simulink model "NDI"  (R2022a)
settings: Solver=ode4  StartTime=0  StopTime=100  FixedStep=fcs.Ts  RelTol=1e-3
undefined symbols (not defined in the file or in its folder): Aactuator, ac, AeroCoeff, ControlAllocation, DUmax, DUmin, EngineTable, F, fcs, ft, g, hground, IC, kg, LandingGear, Light, m, MIL, Mode_deflection_aileron, Mode_deflection_elevator, Mode_deflection_rudder, Mode_deflection_TVC_y, Mode_deflection_TVC_z, N, Ninv_2nozzle, Ninv_no_nozzle, PIController, s, Sensor, sigbuilder_block, slug, state0, sysID_DAQ, sysID_OBES, Umax_2nozzle, Umax_no_nozzle, Umin_2nozzle, Umin_no_nozzle, WMM2020
libraries: aerolibconvert2 x31, slpidlib x11, simulink x6, sharedutil x4, aerolibatmos2 x3, aerolibwind2 x3, aerolibbdyn x3, aerolibgravity2 x2, sharedtransform x1
(part 3 of 13)

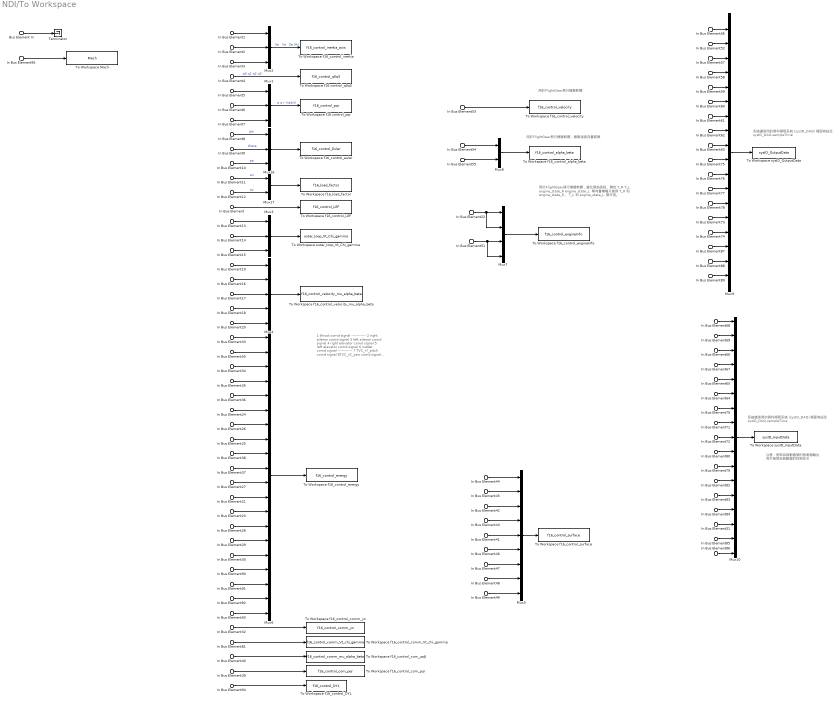
== system NDI/To Workspace ==
  note: 系統識別用的資料擷取系統 (sysID_DAQ)
      | 裡面有設定 sysID_DAQ.sampleTime
  note: 1 thrust comd signal
      | -----------
      | 2 right aileron comd signal
      | 3 left aileron comd signal
      | 4 right elevator comd signal
      | 5 left elevator comd signal
      | 6 rudder comd signal
      | -----------
      | 7 TVC_rY_pitch comd signal
      | 8TVC_rZ_yaw comd signal
      | 9 TVC_lY_pitch comd signal
      | 10TVC_lZ_yaw comd signal
      |
      | 11 thrust signal
      | -----------
      | 12 right aileron signal
      | 13 left aileron signal
      | 14 right elevator signal
      | 15 left elevator signal
      | 16 rudder signal
      | -----------
      | 17 TVC_rY_pitch signal
      | 18 TVC_rZ_yaw signal
      | 19 TVC_lY_pitch signal
      | 20 TVC_lZ_yaw signal
  note: 用於FlightGear飛行模擬軟體
  note: 用於FlightGear飛行模擬軟體，繪製速度向量箭頭
  note: 用於FlightGear飛行模擬軟體，變化尾焰長短、顏色
      | T_R
      | T_L
      | engine_state_R
      | engine_state_L
      |
      | 單向量噴嘴只使用 T_R 和 engine_state_R。
      | T_L 和 engine_state_L 無作用。
  note: 注意：是取自致動器號的感測器輸出
      | 而不是取自致動器的控制命令
  note: 系統識別用的資料擷取系統 (sysID_DAQ)
      | 裡面有設定 sysID_DAQ.sampleTime
  In Bus Element1 : Inport  PortName=PlantData  Element=npos
  In Bus Element2 : Inport  PortName=PlantData  Element=epos
  In Bus Element3 : Inport  PortName=PlantData  Element=altitude
  In Bus Element4 : Inport  PortName=PlantData  Element=q0q1q2q3
  In Bus Element5 : Inport  PortName=PlantData  Element=p
  In Bus Element61 : Inport  PortName=PlantData  Element=p
  In Bus Element6 : Inport  PortName=PlantData  Element=q
  In Bus Element62 : Inport  PortName=PlantData  Element=q
  In Bus Element7 : Inport  PortName=PlantData  Element=r
  In Bus Element63 : Inport  PortName=PlantData  Element=r
  In Bus Element8 : Inport  PortName=PlantData  Element=phi
  In Bus Element58 : Inport  PortName=PlantData  Element=phi
  In Bus Element9 : Inport  PortName=PlantData  Element=theta
  In Bus Element59 : Inport  PortName=PlantData  Element=theta
  In Bus Element10 : Inport  PortName=PlantData  Element=psi
  In Bus Element60 : Inport  PortName=PlantData  Element=psi
  In Bus Element11 : Inport  PortName=PlantData  Element=an
  In Bus Element12 : Inport  PortName=PlantData  Element=ay
  In Bus Element : Inport  PortName=PlantData  Element=AeroActBus.LEF_deg
  In Bus Element80 : Inport  PortName=PlantData  Element=AeroActBus.LEF_deg
  In Bus Element30 : Inport  PortName=PlantData  Element=AeroActBus.Rudder_deg
  In Bus Element41 : Inport  PortName=PlantData  Element=AeroActBus.Rudder_deg
  In Bus Element65 : Inport  PortName=PlantData  Element=AeroActBus.Rudder_deg
  In Bus Element21 : Inport  PortName=PlantData  Element=AeroActBus.right Aileron_deg
  In Bus Element42 : Inport  PortName=PlantData  Element=AeroActBus.right Aileron_deg
  In Bus Element66 : Inport  PortName=PlantData  Element=AeroActBus.right Aileron_deg
  In Bus Element23 : Inport  PortName=PlantData  Element=AeroActBus.left Aileron_deg
  In Bus Element43 : Inport  PortName=PlantData  Element=AeroActBus.left Aileron_deg
  In Bus Element67 : Inport  PortName=PlantData  Element=AeroActBus.left Aileron_deg
  In Bus Element28 : Inport  PortName=PlantData  Element=AeroActBus.right Elevator_deg
  In Bus Element44 : Inport  PortName=PlantData  Element=AeroActBus.right Elevator_deg
  In Bus Element68 : Inport  PortName=PlantData  Element=AeroActBus.right Elevator_deg
  In Bus Element29 : Inport  PortName=PlantData  Element=AeroActBus.left Elevator_deg
  In Bus Element45 : Inport  PortName=PlantData  Element=AeroActBus.left Elevator_deg
  In Bus Element69 : Inport  PortName=PlantData  Element=AeroActBus.left Elevator_deg
  In Bus Element79 : Inport  PortName=PlantData  Element=AeroActBus.SB_deg
  In Bus Element{13,19,53,56} (4 alike) : Inport  PortName=PlantData  Element=Vt
  In Bus Element14 : Inport  PortName=PlantData  Element=chi
  In Bus Element88 : Inport  PortName=PlantData  Element=chi
  In Bus Element15 : Inport  PortName=PlantData  Element=gamma
  In Bus Element20 : Inport  PortName=PlantData  Element=gamma
  In Bus Element89 : Inport  PortName=PlantData  Element=gamma
  In Bus Element16 : Inport  PortName=PlantData  Element=alpha
  In Bus Element54 : Inport  PortName=PlantData  Element=alpha
  In Bus Element52 : Inport  PortName=PlantData  Element=alpha
  In Bus Element17 : Inport  PortName=PlantData  Element=beta
  In Bus Element55 : Inport  PortName=PlantData  Element=beta
  In Bus Element57 : Inport  PortName=PlantData  Element=beta
  In Bus Element18 : Inport  PortName=PlantData  Element=mu
  In Bus Element87 : Inport  PortName=PlantData  Element=mu
  In Bus Element33 : Inport  PortName=PlantData  Element=fadec_cmd.thrust
  In Bus Element25 : Inport  PortName=PlantData  Element=fadec_cmd.TVC_rz
  In Bus Element26 : Inport  PortName=PlantData  Element=fadec_cmd.TVC_ry
  In Bus Element37 : Inport  PortName=PlantData  Element=fadec_cmd.TVC_lz
  In Bus Element38 : Inport  PortName=PlantData  Element=fadec_cmd.TVC_ly
  In Bus Element24 : Inport  PortName=PlantData  Element=fcs_cmd.rudder
  In Bus Element34 : Inport  PortName=PlantData  Element=fcs_cmd.left aileron
  In Bus Element35 : Inport  PortName=PlantData  Element=fcs_cmd.right elevator
  In Bus Element36 : Inport  PortName=PlantData  Element=fcs_cmd.left elevator
  In Bus Element50 : Inport  PortName=PlantData  Element=fcs_cmd.right aileron
  In Bus Element27 : Inport  PortName=PlantData  Element=PropBus.T
  In Bus Element22 : Inport  PortName=PlantData  Element=PropBus.T
  In Bus Element51 : Inport  PortName=PlantData  Element=PropBus.engine_state
  In Bus Element82 : Inport  PortName=PlantData  Element=PropBus.Tx
  In Bus Element83 : Inport  PortName=PlantData  Element=PropBus.Ty
  In Bus Element84 : Inport  PortName=PlantData  Element=PropBus.Tz
  In Bus Element73 : Inport  PortName=PlantData  Element=ay_offset
  In Bus Element74 : Inport  PortName=PlantData  Element=az_offset
  In Bus Element75 : Inport  PortName=PlantData  Element=p_dot
  In Bus Element76 : Inport  PortName=PlantData  Element=q_dot
  In Bus Element77 : Inport  PortName=PlantData  Element=r_dot
  In Bus Element85 : Inport  PortName=PlantData  Element=f
  In Bus Element86 : Inport  PortName=PlantData  Element=N
  In Bus Element90 : Inport  PortName=PlantData  Element=PropActBus.TVC_ry_pitch_deg
  In Bus Element46 : Inport  PortName=PlantData  Element=PropActBus.TVC_ry_pitch_deg
  In Bus Element64 : Inport  PortName=PlantData  Element=PropActBus.TVC_ry_pitch_deg
  In Bus Element91 : Inport  PortName=PlantData  Element=PropActBus.TVC_rz_yaw_deg
  In Bus Element47 : Inport  PortName=PlantData  Element=PropActBus.TVC_rz_yaw_deg
  In Bus Element70 : Inport  PortName=PlantData  Element=PropActBus.TVC_rz_yaw_deg
  In Bus Element92 : Inport  PortName=PlantData  Element=PropActBus.TVC_ly_pitch_deg
  In Bus Element48 : Inport  PortName=PlantData  Element=PropActBus.TVC_ly_pitch_deg
  In Bus Element71 : Inport  PortName=PlantData  Element=PropActBus.TVC_ly_pitch_deg
  In Bus Element93 : Inport  PortName=PlantData  Element=PropActBus.TVC_lz_yaw_deg
  In Bus Element49 : Inport  PortName=PlantData  Element=PropActBus.TVC_lz_yaw_deg
  In Bus Element72 : Inport  PortName=PlantData  Element=PropActBus.TVC_lz_yaw_deg
  In Bus Element78 : Inport  PortName=PlantData  Element=ax_offset
  In Bus Element32 : Inport  PortName=PlantData  Element=LogDataBus.cmd_yz
  In Bus Element39 : Inport  PortName=PlantData  Element=LogDataBus.cmd_pqr
  In Bus Element40 : Inport  PortName=PlantData  Element=LogDataBus.cmd_mu_alpha_beta
  In Bus Element81 : Inport  PortName=PlantData  Element=LogDataBus.cmd_Vt_chi_gamma
  In Bus Element94 : Inport  PortName=PlantData  Element=LogDataBus.drag_sideForce_lift
  Bus Element In : Inport  Port=2  PortName=EnvData
  In Bus Element31 : Inport  Port=2  PortName=EnvData  Element=qbar
  In Bus Element95 : Inport  Port=2  PortName=EnvData  Element=Mach
  Mux{1..3,16} (4 alike) : Mux  Inputs=3
  Mux10 : Mux  Inputs=17
  Mux17 : Mux  Inputs=2
  Mux4 : Mux  Inputs=5
  Mux5 : Mux  Inputs=9
  Mux6 : Mux  Inputs=20
  Mux7 : Mux
  Mux8 : Mux  Inputs=2
  Mux9 : Mux  Inputs=18
  Terminator : Terminator
  To Workspace Mach : ToWorkspace  VariableName=Mach  SaveFormat=Timeseries  SampleTime=-1
  To Workspace f16 control_pqr : ToWorkspace  VariableName=f16_control_pqr  SaveFormat=Timeseries  SampleTime=-1
  To Workspace f16 control_q0q3 : ToWorkspace  VariableName=f16_control_q0q3  SaveFormat=Timeseries  SampleTime=-1
  To Workspace f16_control_DYL : ToWorkspace  VariableName=f16_control_DYL  SaveFormat=Timeseries  SampleTime=-1
  To Workspace f16_control_LEF : ToWorkspace  VariableName=f16_control_LEF  SaveFormat=Timeseries  SampleTime=-1
  To Workspace f16_control_alpha_beta : ToWorkspace  VariableName=f16_control_alpha_beta  SaveFormat=Timeseries  SampleTime=-1
  To Workspace f16_control_com_pqr : ToWorkspace  VariableName=f16_control_com_pqr  SaveFormat=Timeseries  SampleTime=-1
  To Workspace f16_control_com_μαβ : ToWorkspace  VariableName=f16_control_comm_mu_alpha_beta  SaveFormat=Timeseries  SampleTime=-1
  To Workspace f16_control_comm_Vt_chi_gamma : ToWorkspace  VariableName=f16_control_comm_Vt_chi_gamma  SaveFormat=Timeseries  SampleTime=-1
  To Workspace f16_control_comm_yz : ToWorkspace  VariableName=f16_control_comm_yz  SaveFormat=Timeseries  SampleTime=-1
  To Workspace f16_control_energy : ToWorkspace  VariableName=f16_control_energy  SaveFormat=Timeseries  SampleTime=-1
  To Workspace f16_control_engineInfo : ToWorkspace  VariableName=f16_control_engineInfo  SaveFormat=Timeseries  SampleTime=-1
  To Workspace f16_control_euler : ToWorkspace  VariableName=f16_control_Euler  SaveFormat=Timeseries  SampleTime=-1
  To Workspace f16_control_inertia : ToWorkspace  VariableName=f16_control_inertia_axis  SaveFormat=Timeseries  SampleTime=-1
      settings: Save2DSignal=2-D array (concatenate along first dimension)
  To Workspace f16_control_surface : ToWorkspace  VariableName=f16_control_surface  SaveFormat=Timeseries  SampleTime=-1
  To Workspace f16_control_velocity : ToWorkspace  VariableName=f16_control_velocity  SaveFormat=Timeseries  SampleTime=-1
  To Workspace f16_control_velocity_mu_alpha_beta : ToWorkspace  VariableName=f16_control_velocity_mu_alpha_beta  SaveFormat=Timeseries  SampleTime=-1
  To Workspace f16_load_factor : ToWorkspace  VariableName=f16_load_factor  SaveFormat=Timeseries  SampleTime=-1
  To Workspace outer_loop_Vt_Chi_gamma : ToWorkspace  VariableName=outer_loop_Vt_Chi_gamma  SaveFormat=Timeseries  SampleTime=-1
  To Workspace sysID_InputData : ToWorkspace  VariableName=sysID_InputData  SaveFormat=Timeseries  SampleTime=sysID_DAQ.sampleTime
  To Workspace sysID_OutputData : ToWorkspace  VariableName=sysID_OutputData  SaveFormat=Timeseries  SampleTime=sysID_DAQ.sampleTime
  wires:
  Mux2/1 -> To Workspace f16_control_inertia/1  "Xe   Ye   Ze (ft)"
  Mux16/1 -> To Workspace f16_control_euler/1
  In Bus Element9/1 -> Mux16/2  "theta"
  In Bus Element10/1 -> Mux16/3  "psi"
  In Bus Element4/1 -> To Workspace f16 control_q0q3/1  "q0 q1 q2 q3"
  In Bus Element11/1 -> Mux17/1  "an"
  In Bus Element8/1 -> Mux16/1  "phi"
  Mux17/1 -> To Workspace f16_load_factor/1
  In Bus Element12/1 -> Mux17/2  "ay"
  Mux1/1 -> To Workspace f16 control_pqr/1  "p q r (rad/s)"
  In Bus Element5/1 -> Mux1/1
  In Bus Element6/1 -> Mux1/2
  In Bus Element7/1 -> Mux1/3
  In Bus Element1/1 -> Mux2/1
  In Bus Element2/1 -> Mux2/2
  In Bus Element3/1 -> Mux2/3
  In Bus Element/1 -> To Workspace f16_control_LEF/1
  In Bus Element13/1 -> Mux3/1
  In Bus Element14/1 -> Mux3/2
  In Bus Element15/1 -> Mux3/3
  Mux3/1 -> To Workspace outer_loop_Vt_Chi_gamma/1
  In Bus Element19/1 -> Mux4/1
  In Bus Element16/1 -> Mux4/2
  In Bus Element17/1 -> Mux4/3
  In Bus Element18/1 -> Mux4/4
  In Bus Element20/1 -> Mux4/5
  Mux4/1 -> To Workspace f16_control_velocity_mu_alpha_beta/1
  Mux6/1 -> To Workspace f16_control_energy/1
  Bus Element In/1 -> Terminator/1
  In Bus Element33/1 -> Mux6/1
  In Bus Element50/1 -> Mux6/2
  In Bus Element34/1 -> Mux6/3
  In Bus Element35/1 -> Mux6/4
  In Bus Element36/1 -> Mux6/5
  In Bus Element24/1 -> Mux6/6
  In Bus Element27/1 -> Mux6/11
  In Bus Element21/1 -> Mux6/12
  In Bus Element23/1 -> Mux6/13
  In Bus Element28/1 -> Mux6/14
  In Bus Element29/1 -> Mux6/15
  In Bus Element30/1 -> Mux6/16
  In Bus Element90/1 -> Mux6/17
  In Bus Element91/1 -> Mux6/18
  In Bus Element92/1 -> Mux6/19
  In Bus Element93/1 -> Mux6/20
  In Bus Element41/1 -> Mux5/5
  In Bus Element47/1 -> Mux5/7
  In Bus Element49/1 -> Mux5/9
  In Bus Element48/1 -> Mux5/8
  In Bus Element46/1 -> Mux5/6
  In Bus Element44/1 -> Mux5/1
  In Bus Element45/1 -> Mux5/2
  In Bus Element42/1 -> Mux5/3
  In Bus Element43/1 -> Mux5/4
  Mux5/1 -> To Workspace f16_control_surface/1
  In Bus Element26/1 -> Mux6/7
  In Bus Element25/1 -> Mux6/8
  In Bus Element38/1 -> Mux6/9
  In Bus Element37/1 -> Mux6/10
  Mux8/1 -> To Workspace f16_control_alpha_beta/1
  In Bus Element53/1 -> To Workspace f16_control_velocity/1
  In Bus Element55/1 -> Mux8/2
  In Bus Element54/1 -> Mux8/1
  Mux7/1 -> To Workspace f16_control_engineInfo/1
  In Bus Element22/1 -> Mux7/2, Mux7/1
  In Bus Element51/1 -> Mux7/4, Mux7/3
  In Bus Element78/1 -> Mux9/13
  In Bus Element65/1 -> Mux10/5
  In Bus Element75/1 -> Mux9/10
  In Bus Element80/1 -> Mux10/10
  In Bus Element52/1 -> Mux9/2
  In Bus Element79/1 -> Mux10/11
  In Bus Element59/1 -> Mux9/5
  In Bus Element62/1 -> Mux9/8
  In Bus Element83/1 -> Mux10/13
  In Bus Element73/1 -> Mux9/14
  In Bus Element71/1 -> Mux10/8
  In Bus Element60/1 -> Mux9/6
  In Bus Element61/1 -> Mux9/7
  In Bus Element68/1 -> Mux10/1
  In Bus Element77/1 -> Mux9/12
  In Bus Element66/1 -> Mux10/3
  In Bus Element72/1 -> Mux10/9
  In Bus Element69/1 -> Mux10/2
  In Bus Element70/1 -> Mux10/7
  In Bus Element63/1 -> Mux9/9
  In Bus Element58/1 -> Mux9/4
  In Bus Element57/1 -> Mux9/3
  In Bus Element86/1 -> Mux10/17
  In Bus Element67/1 -> Mux10/4
  In Bus Element88/1 -> Mux9/17
  In Bus Element85/1 -> Mux10/16
  In Bus Element76/1 -> Mux9/11
  In Bus Element84/1 -> Mux10/14
  In Bus Element31/1 -> Mux10/15
  In Bus Element82/1 -> Mux10/12
  In Bus Element87/1 -> Mux9/16
  In Bus Element74/1 -> Mux9/15
  In Bus Element89/1 -> Mux9/18
  In Bus Element64/1 -> Mux10/6
  Mux10/1 -> To Workspace sysID_InputData/1
  In Bus Element56/1 -> Mux9/1
  Mux9/1 -> To Workspace sysID_OutputData/1
  In Bus Element94/1 -> To Workspace f16_control_DYL/1
  In Bus Element81/1 -> To Workspace f16_control_comm_Vt_chi_gamma/1
  In Bus Element32/1 -> To Workspace f16_control_comm_yz/1
  In Bus Element40/1 -> To Workspace f16_control_com_μαβ/1
  In Bus Element39/1 -> To Workspace f16_control_com_pqr/1
  In Bus Element95/1 -> To Workspace Mach/1

== system NDI/Environment/Dynamic Pressure ==
  Vt : Inport
  rho : Inport  Port=2
  1/2rhoV^2 : Gain  Gain=1/2  SaturateOnIntegerOverflow=on  OutDataTypeStr=Inherit: Same as input  ParamDataTypeStr=Inherit: Same as input
  Product2 : Product  InputSameDT=on  SaturateOnIntegerOverflow=on  OutDataTypeStr=Inherit: Same as first input
  Square : Math  Operator=square  SignedPower=on
  qbar : Outport
  wires:
  rho/1 -> Product2/2
  Square/1 -> Product2/1
  1/2rhoV^2/1 -> qbar/1
  Product2/1 -> 1/2rhoV^2/1
  Vt/1 -> Square/1

== system NDI/Environment/ISP  ==
  note: 1 T
      | 2 a (Speed of sound)
      | 3 P
      | 4 rho
      | 5 g
      | 6 mu (Coefficient of viscosity)
  h(m) : Inport
  Demux : Demux  Outputs=[1,1,1,1,1,1]
      settings: DisplayOption=none
  MATLAB Function : MATLAB Function  TreatAsAtomicUnit=on
  end8 : Terminator
  end9 : Terminator
  T (K) : Outport  VectorParamsAs1DForOutWhenUnconnected=off
  a (m/s) : Outport  Port=2  VectorParamsAs1DForOutWhenUnconnected=off
  P (HPa) : Outport  Port=3  VectorParamsAs1DForOutWhenUnconnected=off
  rho (kg/m^3) : Outport  Port=4  VectorParamsAs1DForOutWhenUnconnected=off
  wires:
  MATLAB Function/1(ISP_output) -> Demux/1
  h(m)/1 -> MATLAB Function/1(h)
  Demux/4 -> rho (kg/m^3)/1  "rho(kg/m^3)"
  Demux/2 -> a (m/s)/1  "a(m/s)"
  Demux/1 -> T (K)/1  "T(K)"
  Demux/5 -> end8/1  "g (m/s^2)"
  Demux/6 -> end9/1  "mu"
  Demux/3 -> P (HPa)/1  "P(Pa)"

== system NDI/Environment/Mach Number ==
  Vt : Inport
  a : Inport  Port=2
  Product1 : Product  Inputs=*/  InputSameDT=on  SaturateOnIntegerOverflow=on  OutDataTypeStr=Inherit: Same as first input
  Mach : Outport  Unit=1  VectorParamsAs1DForOutWhenUnconnected=off
  wires:
  Vt/1 -> Product1/1
  a/1 -> Product1/2
  Product1/1 -> Mach/1

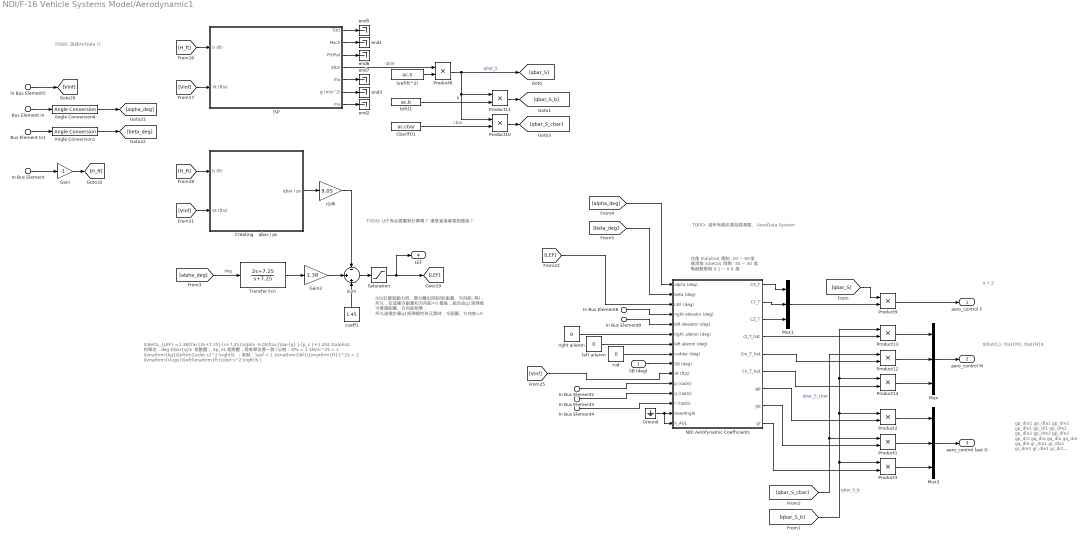
== system NDI/F-16 Vehicle Systems Model/Aerodynamic1 ==
  note: NDI計算氣動力時，要分離出控制項(副翼、方向舵..等)，
      | 所以，在這裡令副翼和方向舵=0
      | 最後，組合成g1矩陣後 才會跟副翼、方向舵相乘，
      | 所以這裡計算g1矩陣裡的各元素時，令副翼、方向舵=0
  note: TODO: LEF有必要重新計算嗎？
      | 還是直接拿感測器值？
  note: X
      | Y
      | Z
  note: $\delta_{LEF} =1.38\frac{2s+7.25}{s+7.25}\alpha -9.05\frac{\bar{q} }{p_s }+1.45$
      | $\alpha$ 的單位：deg
      | $\bar{q}$ 是動壓， $p_s$ 是靜壓，兩者單位要一致 (公制：1Pa = 1 $N/m^2$ = 1 $\mathrm{kg}/\left(m{\cdot s}^2 \right)$ ；英制：1psf = 1 $\mathrm{lbf}/{\mathrm{ft}}^2$ = 1 $\mathrm{slugs}/\left(\mathrm{ft}\cdot s^2 \right)$ )
  note: $\hat{L}, \hat{M}, \hat{N}$
  note: TODO: 這所有資訊源自感測器、
      | AeroData System
  note: TODO: 改成AirData !?
  note: 攻角 $\alpha$ 限制 -20 ~ 90度
      | 側滑角 $\beta$ 限制 -30 ~ 30 度
      | 馬赫數限制 0.1 ~ 0.6 度
  note: gp_dra1
      | gp_dla1
      | gp_dre1
      | gp_dle1
      | gp_dr1
      | gp_dra2
      | gp_dla2
      | gp_dre2
      | gp_dle2
      | gp_dr2
      |
      | gq_dra
      | gq_dla
      | gq_dre
      | gq_dle
      |
      | gr_dra1
      | gr_dla1
      | gr_dre1
      | gr_dle1
      | gr_dr1
      | gr_dra2
      | gr_dla2
      | gr_dre2
      | gr_dle2
      | gr_dr2
  SB (deg) : Inport  Unit=deg
  In Bus Element : Inport  Port=2  PortName=PlantData  Element=altitude
  In Bus Element8 : Inport  Port=2  PortName=PlantData  Element=AeroActBus.right Elevator_deg
  In Bus Element9 : Inport  Port=2  PortName=PlantData  Element=AeroActBus.left Elevator_deg
  In Bus Element2 : Inport  Port=2  PortName=PlantData  Element=p
  In Bus Element3 : Inport  Port=2  PortName=PlantData  Element=q
  In Bus Element4 : Inport  Port=2  PortName=PlantData  Element=r
  In Bus Element5 : Inport  Port=2  PortName=PlantData  Element=Vt
  Bus Element In : Inport  Port=3  PortName=AirData  Element=alpha
  Bus Element In1 : Inport  Port=3  PortName=AirData  Element=beta
  Angle Conversion1 : aerolibconvert2/Angle Conversion  IU=rad  OU=deg
  Angle Conversion4 : aerolibconvert2/Angle Conversion  IU=rad  OU=deg
  Cbar(ft)1 : Constant  Value=ac.cbar
  Creating    qbar / ps : Subsystem
  Gain : Gain  Gain=-1
  Gain2 : Gain  Gain=1.38  SaturateOnIntegerOverflow=on  OutDataTypeStr=Inherit: Same as input  ParamDataTypeStr=Inherit: Same as input
  Ground : Ground
  "ISP " : Subsystem
  Mux : Mux  Inputs=3
  Mux1 : Mux  Inputs=3
  Mux3 : Mux  Inputs=3
  NDI Aerofynamic Coefficients : Subsystem
  Product{1..3,6,9..14} (10 alike) : Product
  Saturation : Saturate  UpperLimit=Aactuator.LEF.AngleLimitUpper  LowerLimit=Aactuator.LEF.AngleLimitLower
  Sref(ft^2) : Constant  Value=ac.S
  Sum : Sum  Inputs=-|+|+  InputSameDT=on  SaturateOnIntegerOverflow=on  OutDataTypeStr=Inherit: Same as first input
  Transfer Fcn : TransferFcn  Numerator=[2 7.25]  Denominator=[1 7.25]
  b(ft)1 : Constant  Value=ac.b
  coeff1 : Constant  Value=1.45
  end{1..3,5..7} (6 alike) : Terminator
  left aileron : Constant  Value=0
  r2d6 : Gain  Gain=9.05  SaturateOnIntegerOverflow=on  OutDataTypeStr=Inherit: Same as input  ParamDataTypeStr=Inherit: Same as input
  right aileron : Constant  Value=0
  rud : Constant  Value=0
  aero_control F : Outport  VectorParamsAs1DForOutWhenUnconnected=off
  aero_control M : Outport  Port=2  VectorParamsAs1DForOutWhenUnconnected=off
  aero_control fast G : Outport  Port=3  VectorParamsAs1DForOutWhenUnconnected=off
  LEF : Outport  Port=4
  wires:
  [Vinf] -> "ISP "/2(Vt (ft/s))
  "ISP "/2("Mach ") -> end1/1
  "ISP "/7(mu) -> end2/1
  "ISP "/6(g (m/s^2)) -> end3/1
  "ISP "/5(rho) -> end7/1
  "ISP "/4("qbar ") -> Product6/1  "qbar"
  "ISP "/3(P(HPa)) -> end6/1
  "ISP "/1(T(K)) -> end5/1
  r2d6/1 -> Sum/1
  Creating    qbar / ps/1(qbar / ps) -> r2d6/1
  [alpha_deg] -> Transfer Fcn/1  "deg"
  [Vinf] -> Creating    qbar / ps/2(Vt (ft/s))
  coeff1/1 -> Sum/3
  [H_ft] -> Creating    qbar / ps/1(h (ft))
  [H_ft] -> "ISP "/1(h (ft))
  Sum/1 -> Saturation/1
  Saturation/1 -> LEF/1, [LEF]
  Transfer Fcn/1 -> Gain2/1
  In Bus Element/1 -> Gain/1
  Gain/1 -> [H_ft]
  Cbar(ft)1/1 -> Product10/2  "cbar"
  b(ft)1/1 -> Product11/2  "b"
  Sref(ft^2)/1 -> Product6/2
  Product10/1 -> [qbar_S_cbar]
  Product6/1 -> Product11/1, Product10/1, [qbar_S]  "qbar_S"
  Product11/1 -> [qbar_S_b]
  [qbar_S] -> Product9/1
  Product9/1 -> aero_control F/1
  Product12/1 -> Mux/2
  Product13/1 -> Mux/1
  Product14/1 -> Mux/3
  Mux/1 -> aero_control M/1
  NDI Aerofynamic Coefficients/4(Cl_T_hat) -> Product13/2
  NDI Aerofynamic Coefficients/5(Cm_T_hat) -> Product12/2
  NDI Aerofynamic Coefficients/6(Cn_T_hat) -> Product14/2
  NDI Aerofynamic Coefficients/1(CX_T) -> Mux1/1
  NDI Aerofynamic Coefficients/2(CY_T) -> Mux1/2
  NDI Aerofynamic Coefficients/3(CZ_T) -> Mux1/3
  Mux1/1 -> Product9/2
  [qbar_S_b] -> Product13/1, Product14/1, Product2/1, Product3/1  "qbar_S_b"
  Product3/1 -> Mux3/3
  Product1/1 -> Mux3/2
  Product2/1 -> Mux3/1
  NDI Aerofynamic Coefficients/7(gp) -> Product2/2
  [qbar_S_cbar] -> Product12/1, Product1/1  "qbar_S_cbar"
  NDI Aerofynamic Coefficients/9(gr) -> Product3/2
  NDI Aerofynamic Coefficients/8(gq) -> Product1/2
  Mux3/1 -> aero_control fast G/1
  [Vinf] -> NDI Aerofynamic Coefficients/10(Vt (ft/s))
  SB (deg)/1 -> NDI Aerofynamic Coefficients/9(SB (deg))
  [LEF] -> NDI Aerofynamic Coefficients/3(LEF (deg))
  [beta_deg] -> NDI Aerofynamic Coefficients/2(beta (deg))
  [alpha_deg] -> NDI Aerofynamic Coefficients/1(alpha (deg))
  In Bus Element2/1 -> NDI Aerofynamic Coefficients/11(p (rad/s))
  In Bus Element3/1 -> NDI Aerofynamic Coefficients/12(q (rad/s))
  In Bus Element4/1 -> NDI Aerofynamic Coefficients/13(r (rad/s))
  Ground/1 -> NDI Aerofynamic Coefficients/14(GearAngle), NDI Aerofynamic Coefficients/15(h_AGL)
  Gain2/1 -> Sum/2
  Bus Element In/1 -> Angle Conversion4/1
  Angle Conversion4/1 -> [alpha_deg]
  Angle Conversion1/1 -> [beta_deg]
  Bus Element In1/1 -> Angle Conversion1/1
  In Bus Element5/1 -> [Vinf]
  In Bus Element8/1 -> NDI Aerofynamic Coefficients/4(right elevator (deg))
  In Bus Element9/1 -> NDI Aerofynamic Coefficients/5(left elevator (deg))
  right aileron/1 -> NDI Aerofynamic Coefficients/6(right alieron (deg))
  left aileron/1 -> NDI Aerofynamic Coefficients/7(left alieron (deg))
  rud/1 -> NDI Aerofynamic Coefficients/8(rudder (deg))

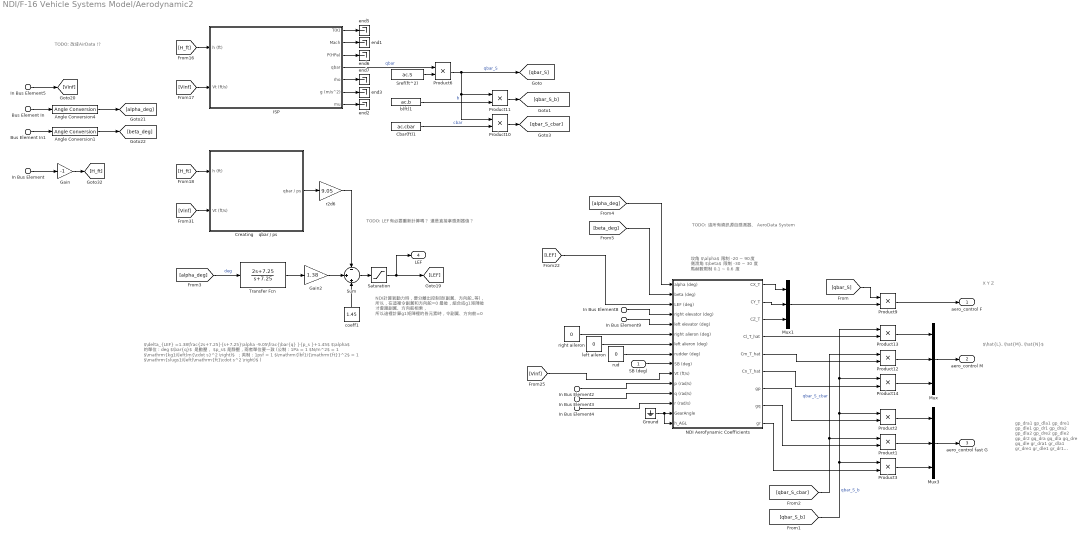
== system NDI/F-16 Vehicle Systems Model/Aerodynamic2 ==
  note: NDI計算氣動力時，要分離出控制項(副翼、方向舵..等)，
      | 所以，在這裡令副翼和方向舵=0
      | 最後，組合成g1矩陣後 才會跟副翼、方向舵相乘，
      | 所以這裡計算g1矩陣裡的各元素時，令副翼、方向舵=0
  note: TODO: LEF有必要重新計算嗎？
      | 還是直接拿感測器值？
  note: X
      | Y
      | Z
  note: $\delta_{LEF} =1.38\frac{2s+7.25}{s+7.25}\alpha -9.05\frac{\bar{q} }{p_s }+1.45$
      | $\alpha$ 的單位：deg
      | $\bar{q}$ 是動壓， $p_s$ 是靜壓，兩者單位要一致 (公制：1Pa = 1 $N/m^2$ = 1 $\mathrm{kg}/\left(m{\cdot s}^2 \right)$ ；英制：1psf = 1 $\mathrm{lbf}/{\mathrm{ft}}^2$ = 1 $\mathrm{slugs}/\left(\mathrm{ft}\cdot s^2 \right)$ )
  note: $\hat{L}, \hat{M}, \hat{N}$
  note: TODO: 這所有資訊源自感測器、
      | AeroData System
  note: TODO: 改成AirData !?
  note: 攻角 $\alpha$ 限制 -20 ~ 90度
      | 側滑角 $\beta$ 限制 -30 ~ 30 度
      | 馬赫數限制 0.1 ~ 0.6 度
  note: gp_dra1
      | gp_dla1
      | gp_dre1
      | gp_dle1
      | gp_dr1
      | gp_dra2
      | gp_dla2
      | gp_dre2
      | gp_dle2
      | gp_dr2
      |
      | gq_dra
      | gq_dla
      | gq_dre
      | gq_dle
      |
      | gr_dra1
      | gr_dla1
      | gr_dre1
      | gr_dle1
      | gr_dr1
      | gr_dra2
      | gr_dla2
      | gr_dre2
      | gr_dle2
      | gr_dr2
  SB (deg) : Inport  Unit=deg
  In Bus Element : Inport  Port=2  PortName=PlantData  Element=altitude
  In Bus Element8 : Inport  Port=2  PortName=PlantData  Element=AeroActBus.right Elevator_deg
  In Bus Element9 : Inport  Port=2  PortName=PlantData  Element=AeroActBus.left Elevator_deg
  In Bus Element2 : Inport  Port=2  PortName=PlantData  Element=p
  In Bus Element3 : Inport  Port=2  PortName=PlantData  Element=q
  In Bus Element4 : Inport  Port=2  PortName=PlantData  Element=r
  In Bus Element5 : Inport  Port=2  PortName=PlantData  Element=Vt
  Bus Element In : Inport  Port=3  PortName=AirData  Element=alpha
  Bus Element In1 : Inport  Port=3  PortName=AirData  Element=beta
  Angle Conversion1 : aerolibconvert2/Angle Conversion  IU=rad  OU=deg
  Angle Conversion4 : aerolibconvert2/Angle Conversion  IU=rad  OU=deg
  Cbar(ft)1 : Constant  Value=ac.cbar
  Creating    qbar / ps : Subsystem
  Gain : Gain  Gain=-1
  Gain2 : Gain  Gain=1.38  SaturateOnIntegerOverflow=on  OutDataTypeStr=Inherit: Same as input  ParamDataTypeStr=Inherit: Same as input
  Ground : Ground
  "ISP " : Subsystem
  Mux : Mux  Inputs=3
  Mux1 : Mux  Inputs=3
  Mux3 : Mux  Inputs=3
  NDI Aerofynamic Coefficients : Subsystem
  Product{1..3,6,9..14} (10 alike) : Product
  Saturation : Saturate  UpperLimit=Aactuator.LEF.AngleLimitUpper  LowerLimit=Aactuator.LEF.AngleLimitLower
  Sref(ft^2) : Constant  Value=ac.S
  Sum : Sum  Inputs=-|+|+  InputSameDT=on  SaturateOnIntegerOverflow=on  OutDataTypeStr=Inherit: Same as first input
  Transfer Fcn : TransferFcn  Numerator=[2 7.25]  Denominator=[1 7.25]
  b(ft)1 : Constant  Value=ac.b
  coeff1 : Constant  Value=1.45
  end{1..3,5..7} (6 alike) : Terminator
  left aileron : Constant  Value=0
  r2d6 : Gain  Gain=9.05  SaturateOnIntegerOverflow=on  OutDataTypeStr=Inherit: Same as input  ParamDataTypeStr=Inherit: Same as input
  right aileron : Constant  Value=0
  rud : Constant  Value=0
  aero_control F : Outport  VectorParamsAs1DForOutWhenUnconnected=off
  aero_control M : Outport  Port=2  VectorParamsAs1DForOutWhenUnconnected=off
  aero_control fast G : Outport  Port=3  VectorParamsAs1DForOutWhenUnconnected=off
  LEF : Outport  Port=4
  wires:
  [Vinf] -> "ISP "/2(Vt (ft/s))
  "ISP "/2("Mach ") -> end1/1
  "ISP "/7(mu) -> end2/1
  "ISP "/6(g (m/s^2)) -> end3/1
  "ISP "/5(rho) -> end7/1
  "ISP "/4("qbar ") -> Product6/1  "qbar"
  "ISP "/3(P(HPa)) -> end6/1
  "ISP "/1(T(K)) -> end5/1
  r2d6/1 -> Sum/1
  Creating    qbar / ps/1(qbar / ps) -> r2d6/1
  [alpha_deg] -> Transfer Fcn/1  "deg"
  [Vinf] -> Creating    qbar / ps/2(Vt (ft/s))
  coeff1/1 -> Sum/3
  [H_ft] -> Creating    qbar / ps/1(h (ft))
  [H_ft] -> "ISP "/1(h (ft))
  Sum/1 -> Saturation/1
  Saturation/1 -> LEF/1, [LEF]
  Transfer Fcn/1 -> Gain2/1
  In Bus Element/1 -> Gain/1
  Gain/1 -> [H_ft]
  Cbar(ft)1/1 -> Product10/2  "cbar"
  b(ft)1/1 -> Product11/2  "b"
  Sref(ft^2)/1 -> Product6/2
  Product10/1 -> [qbar_S_cbar]
  Product6/1 -> Product11/1, Product10/1, [qbar_S]  "qbar_S"
  Product11/1 -> [qbar_S_b]
  [qbar_S] -> Product9/1
  Product9/1 -> aero_control F/1
  Product12/1 -> Mux/2
  Product13/1 -> Mux/1
  Product14/1 -> Mux/3
  Mux/1 -> aero_control M/1
  NDI Aerofynamic Coefficients/4(Cl_T_hat) -> Product13/2
  NDI Aerofynamic Coefficients/5(Cm_T_hat) -> Product12/2
  NDI Aerofynamic Coefficients/6(Cn_T_hat) -> Product14/2
  NDI Aerofynamic Coefficients/1(CX_T) -> Mux1/1
  NDI Aerofynamic Coefficients/2(CY_T) -> Mux1/2
  NDI Aerofynamic Coefficients/3(CZ_T) -> Mux1/3
  Mux1/1 -> Product9/2
  [qbar_S_b] -> Product13/1, Product14/1, Product2/1, Product3/1  "qbar_S_b"
  Product3/1 -> Mux3/3
  Product1/1 -> Mux3/2
  Product2/1 -> Mux3/1
  NDI Aerofynamic Coefficients/7(gp) -> Product2/2
  [qbar_S_cbar] -> Product12/1, Product1/1  "qbar_S_cbar"
  NDI Aerofynamic Coefficients/9(gr) -> Product3/2
  NDI Aerofynamic Coefficients/8(gq) -> Product1/2
  Mux3/1 -> aero_control fast G/1
  [Vinf] -> NDI Aerofynamic Coefficients/10(Vt (ft/s))
  SB (deg)/1 -> NDI Aerofynamic Coefficients/9(SB (deg))
  [LEF] -> NDI Aerofynamic Coefficients/3(LEF (deg))
  [beta_deg] -> NDI Aerofynamic Coefficients/2(beta (deg))
  [alpha_deg] -> NDI Aerofynamic Coefficients/1(alpha (deg))
  In Bus Element2/1 -> NDI Aerofynamic Coefficients/11(p (rad/s))
  In Bus Element3/1 -> NDI Aerofynamic Coefficients/12(q (rad/s))
  In Bus Element4/1 -> NDI Aerofynamic Coefficients/13(r (rad/s))
  Ground/1 -> NDI Aerofynamic Coefficients/14(GearAngle), NDI Aerofynamic Coefficients/15(h_AGL)
  Gain2/1 -> Sum/2
  Bus Element In/1 -> Angle Conversion4/1
  Angle Conversion4/1 -> [alpha_deg]
  Angle Conversion1/1 -> [beta_deg]
  Bus Element In1/1 -> Angle Conversion1/1
  In Bus Element5/1 -> [Vinf]
  In Bus Element8/1 -> NDI Aerofynamic Coefficients/4(right elevator (deg))
  In Bus Element9/1 -> NDI Aerofynamic Coefficients/5(left elevator (deg))
  right aileron/1 -> NDI Aerofynamic Coefficients/6(right alieron (deg))
  left aileron/1 -> NDI Aerofynamic Coefficients/7(left alieron (deg))
  rud/1 -> NDI Aerofynamic Coefficients/8(rudder (deg))

== system NDI/F-16 Vehicle Systems Model/Iteration Algorithm V chi gamma ==
  note: TODO: 這有必要嗎？
      | 設定限制範圍錯誤似乎會造成計算問題，第0秒模擬失敗
  note: $\mu_c ={\mathrm{tan}}^{-1} {\left(\frac{mV_T {\chi^˙ }_{des} \mathrm{cos}\gamma-f\mathrm{sin}\chi }{mV_T {\gamma^˙ }_{des} +mg\mathrm{cos}\gamma-N\mathrm{cos}\gamma-f\mathrm{cos}\chi\mathrm{sin}\gamma }\right)}$
  note: $\alpha_c ={\mathrm{tan}}^{-1} {\left(\frac{-L+mV_T {\chi^˙ }_{des} \mathrm{cos}\gamma \mathrm{sin}\mu_c +mV_T {\gamma^˙ }_{des} \mathrm{cos}\mu_c +mg\mathrm{cos}\gamma \mathrm{cos}\mu_c-N\mathrm{cos}\mu_c\mathrm{cos}\gamma-f(\mathrm{sin}\mu_c\mathrm{sin}\chi+\mathrm{cos}\mu_c\mathrm{cos}\chi\mathrm{sin}\gamma) }{m{\dot{V} }_{T_{des} } +D+mg\mathrm{sin}\gamma-N\mathrm{sin}\gamma+f\mathrm{cos}\chi\mathrm{sin}\gamma }\right)}$
  note: $T_c =\frac{1}{\mathrm{cos}\alpha_c }{\left(m{\dot{V} }_{T_{des} } +D+mg\mathrm{sin}\gamma-N\mathrm{sin}\gamma+f\mathrm{cos}\chi\mathrm{sin}\gamma \right)}$
  note: m
  note: chi
  note: f,0,N
  note: chi
  note: f,0,N
  note: chi
  note: f,0,N
  alpha_c : Inport
  aero F : Inport  Port=2
  Vt,chi,gamma dot desire : Inport  Port=3
  beta_cmd : Inport  Port=4
  LGxyz : Inport  Port=5
  gravity : Inport  Port=6
  In Bus Element4 : Inport  Port=7  PortName=AirData  Element=Vt
  In Bus Element5 : Inport  Port=7  PortName=AirData  Element=gamma
  In Bus Element1 : Inport  Port=8  PortName=PlantData  Element=chi
  Drag_c : Fcn  Expr=-u(4)*cos(u(2))*cos(u(3))-u(5)*sin(u(3))-u(6)*sin(u(2))*cos(u(3))
  Lift_c : Fcn  Expr=u(4)*sin(u(2))-u(6)*cos(u(2))
  Mux : Mux  Inputs=7
  Mux1 : Mux
  Mux2 : Mux  Inputs=7
  Mux{3..6} (4 alike) : Mux  Inputs=2
  Mux7 : Mux  Inputs=7
  Saturation : Saturate  UpperLimit=deg2rad(90)  LowerLimit=deg2rad(-20)
  Thrust_c function : Fcn  Expr=(u(8)*u(1)+u(6)+u(8)*u(9)*sin(u(5))+u(14)*sin(u(5))-u(12)*cos(u(11))*sin(u(5)))/(cos(u(10)))
  To Workspace : ToWorkspace  VariableName=Drag_c_Lift_c  SaveFormat=Timeseries  SampleTime=-1
  alpha_c function : Fcn  Expr=atan2((-u(9)+u(10)*u(6)*cos(u(7))*sin(u(4))*u(2)+u(10)*u(6)*cos(u(4))*u(3)+u(10)*u(11)*cos(u(7))*cos(u(4))+u(15)*cos(u(4))*cos(u(7))+u(13)*(sin(u(4))*sin(u(12))+cos(u(4))*cos(u(12))*sin(u(7)))),(u(10)*u(1)+u(8)+u(10)*u(11)*sin(u(7))+u(15)*sin(u(7))-u(13)*cos(u(12))*sin(u(7))))
  mass (slugs) : Constant  Value=ac.m
  mu_c : Fcn  Expr=atan2((u(7)*u(4)*u(2)*cos(u(5))-u(9)*sin(u(8))),(u(7)*u(4)*u(3)+u(7)*u(6)*cos(u(5))-u(11)*cos(u(5))-u(9)*cos(u(8))*sin(u(5))))
  thrust_command : Outport  VectorParamsAs1DForOutWhenUnconnected=off
  mu_command : Outport  Port=2  VectorParamsAs1DForOutWhenUnconnected=off
  alpha_command : Outport  Port=3  VectorParamsAs1DForOutWhenUnconnected=off
  beta_command : Outport  Port=4  VectorParamsAs1DForOutWhenUnconnected=off
  wires:
  Vt,chi,gamma dot desire/1 -> Mux/1, Mux2/1, Mux7/1  "Vt,chi,gamma dot desire"
  In Bus Element4/1 -> Mux6/1, Mux1/1, Mux/2  "Vt"
  In Bus Element5/1 -> Mux6/2, Mux/3  "gamma"
  Mux/1 -> mu_c/1
  gravity/1 -> Mux5/2, Mux/4  "g"
  mu_c/1 -> Mux4/1, mu_command/1  "mu_c"
  aero F/1 -> Mux1/4  "X,Y,Z"
  beta_cmd/1 -> Mux4/2, Mux1/3, beta_command/1  "beta_c"
  alpha_c/1 -> Mux1/2  "alpha_c"
  Mux1/1 -> Lift_c/1, Drag_c/1
  Drag_c/1 -> Mux3/1  "Drag_c"
  Lift_c/1 -> Mux3/2  "Lift_c"
  Mux3/1 -> To Workspace/1, Mux2/4, Mux7/3  "Drag_c,Lift_c"
  Mux4/1 -> Mux2/2  "mu_c,beta_c"
  mass (slugs)/1 -> Mux/5, Mux5/1  "mass"
  Mux5/1 -> Mux2/5, Mux7/4  "mass,gravity"
  Mux6/1 -> Mux7/2, Mux2/3  "Vt,gamma"
  In Bus Element1/1 -> Mux/6, Mux2/6, Mux7/6
  LGxyz/1 -> Mux/7, Mux7/7, Mux2/7
  Saturation/1 -> alpha_command/1, Mux7/5
  Mux2/1 -> alpha_c function/1  "alpha_c"
  alpha_c function/1 -> Saturation/1  "alpha_c"
  Mux7/1 -> Thrust_c function/1  "thrust_c"
  Thrust_c function/1 -> thrust_command/1  "thrust_c"

== system NDI/F-16 Vehicle Systems Model/Iteration Algorithm Y Z ==
  note: $\chi_c ={\mathrm{sin}}^{-1} {\left(\frac{{\dot{Y} }_{des} }{\sqrt{V_{T_c }^2 -{\dot{Z} }_{des}^2 }}\right)}$
  note: $\gamma_c =-{\mathrm{sin}}^{-1} {\left(\frac{{\dot{Z} }_{des} }{V_{T_c } }\right)}$
  Vc : Inport
  Ydot,Zdot des : Inport  Port=2
  Asin : Trigonometry  Operator=asin
  Asin1 : Trigonometry  Operator=asin
  Demux : Demux  Outputs=2
  Divide : Product  Inputs=*/
  Divide1 : Product  Inputs=*/
  Minus : Sum  Inputs=+-
  Multiply : Gain  Gain=-1
  Square : Math  Operator=square
  Square Root : Sqrt
  Square1 : Math  Operator=square
  chi_c : Outport  VectorParamsAs1DForOutWhenUnconnected=off
  gamma_c : Outport  Port=2  VectorParamsAs1DForOutWhenUnconnected=off
  wires:
  Vc/1 -> Square/1, Divide/2  "Vc"
  Ydot,Zdot des/1 -> Demux/1
  Asin/1 -> Multiply/1
  Divide/1 -> Asin/1
  Demux/2 -> Square1/1, Divide/1  "Z_dot_desire"
  Demux/1 -> Divide1/1  "Y_dot_desire"
  Asin1/1 -> chi_c/1
  Divide1/1 -> Asin1/1
  Square Root/1 -> Divide1/2
  Square/1 -> Minus/1
  Square1/1 -> Minus/2
  Minus/1 -> Square Root/1
  Multiply/1 -> gamma_c/1

== system NDI/F-16 Vehicle Systems Model/Landing_Control ==
  thrust : Inport
  mu_alpha_beta : Inport  Port=2
  In Bus Element : Inport  Port=3  PortName=PlantData  Element=Vt
  In Bus Element44 : Inport  Port=3  PortName=PlantData  Element=LGBus.LeftMain_WOW
  In Bus Element47 : Inport  Port=3  PortName=PlantData  Element=LGBus.RightMain_WOW
  Logical Operator : Logic  AllPortsSameDT=off  OutDataTypeStr=boolean
  Mux8 : Mux  Inputs=3
  Stateflow : Stateflow chart  TreatAsAtomicUnit=on
  Switch : Switch  Criteria=u2 ~= 0  SaturateOnIntegerOverflow=off  InputSameDT=off
  Switch1 : Switch  Criteria=u2 ~= 0  SaturateOnIntegerOverflow=off  InputSameDT=off
  thrust_command : Outport
  mu_alpha_beta_command : Outport  Port=2
  wires:
  Logical Operator/1 -> Switch/2, Switch1/2
  Stateflow/1(T) -> Switch1/1
  Mux8/1 -> Switch/1  "mu alpha beta command (rad)"
  Stateflow/2(mu) -> Mux8/1
  Stateflow/3(alpha) -> Mux8/2
  Stateflow/4(beta) -> Mux8/3
  In Bus Element/1 -> Stateflow/1(Vt)
  In Bus Element47/1 -> Logical Operator/1
  In Bus Element44/1 -> Logical Operator/2
  thrust/1 -> Switch1/3
  mu_alpha_beta/1 -> Switch/3
  Switch1/1 -> thrust_command/1  "thrust"
  Switch/1 -> mu_alpha_beta_command/1
